simulink model "solarSystemsimulation"  (R2025b)
settings: Solver=ode45  StartTime=0.0  StopTime=T_sim  MaxStep=3600  RelTol=1e-3
values from neighbouring files (symbols this model uses):
  P0 = Raw_All(1:3, :) * km2m    [init_file.m]
  V0 = Raw_All(4:6, :) * km2m    [init_file.m]
settings Model: Creator=leupe  LastModifiedBy=leupe

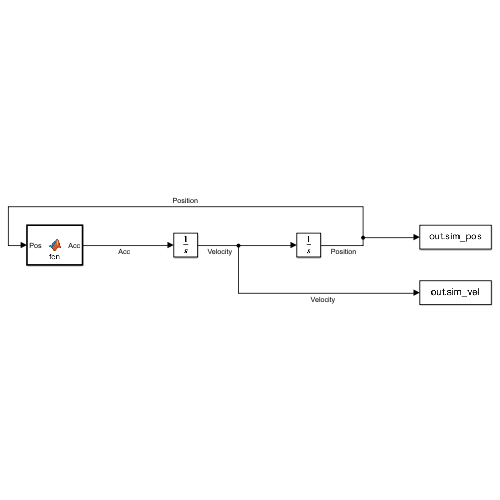
[thumbnail: Simulink's stored preview of the top-level diagram]
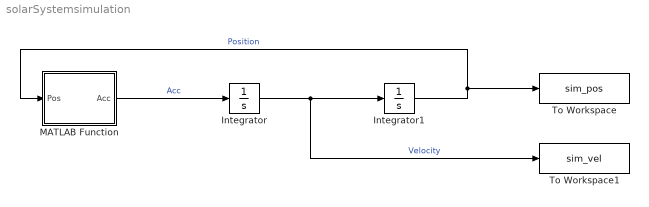
== system solarSystemsimulation ==
  Integrator : Integrator  InitialCondition=V0
  Integrator1 : Integrator  InitialCondition=P0
  MATLAB Function : MATLAB Function  TreatAsAtomicUnit=on
  To Workspace : ToWorkspace  VariableName=sim_pos  SampleTime=-1
  To Workspace1 : ToWorkspace  VariableName=sim_vel  SampleTime=-1
  wires:
  MATLAB Function/1(Acc) -> Integrator/1  "Acc"
  Integrator/1 -> To Workspace1/1, Integrator1/1  "Velocity"
  Integrator1/1 -> MATLAB Function/1(Pos), To Workspace/1  "Position"

== matlab function solarSystemsimulation/MATLAB Function ==
  data: Pos input; Acc output
function Acc = fcn(Pos)
    % Definim parametrii ca fiind externi (din Workspace)
    % M = vector 1x9 (mase), G = constanta gravitationala
    M = [1.98841e30, 3.302e23, 4.8685e24, 6.046e24, 6.417e23, 1.898e27, 5.683e26, 8.681e25, 1.024e26];
    G = 6.6743e-11;
    
    % Initializam acceleratia (3 randuri x 9 coloane)
    Acc = zeros(3, 9);
    N = 9;
    
    for i = 1:N
        for j = 1:N
            if i ~= j
                % Vectorul distanta r_j - r_i
                r_rel = Pos(:, j) - Pos(:, i);
                
                % Distanta scalara (norma)
                dist = sqrt(sum(r_rel.^2));
                
                % Formula gravitatiei: a_i += G * m_j * r_rel / dist^3
                Acc(:, i) = Acc(:, i) + (G * M(j) * r_rel) / (dist^3);
            end
        end
    end
end
